simulink model "Expt_2_1"  (R2018a)
settings: Solver=VariableStepAuto  StartTime=0.0  StopTime=10.0  RelTol=1e-3
settings Model: Creator=HP  LastModifiedBy=HP

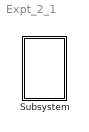
== system Expt_2_1 ==
  Subsystem : Subsystem

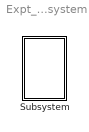
== system Expt_2_1/Subsystem ==
  Subsystem : Subsystem

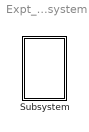
== system Expt_2_1/Subsystem/Subsystem ==
  Subsystem : Subsystem

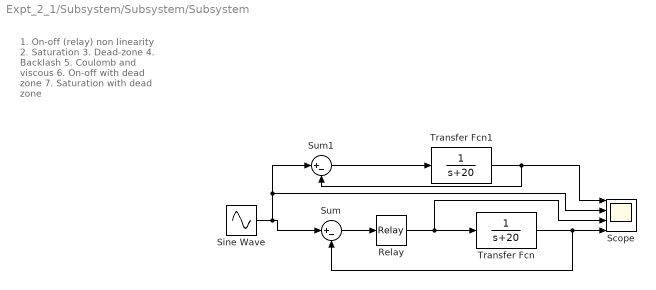
== system Expt_2_1/Subsystem/Subsystem/Subsystem ==
  note: 1. On-off (relay) non linearity
      | 2. Saturation
      | 3. Dead-zone
      | 4. Backlash
      | 5. Coulomb and viscous
      | 6. On-off with dead zone
      | 7. Saturation with dead zone
  Relay : Relay
  Scope : Scope  NumInputPorts=4
  Sine Wave : Sin  SampleTime=0
  Sum : Sum  Inputs=|+-
  Sum1 : Sum  Inputs=|+-
  Transfer Fcn : TransferFcn  Denominator=[1 20]
  Transfer Fcn1 : TransferFcn  Denominator=[1 20]
  wires:
  Sum1/1 -> Transfer Fcn1/1
  Sum/1 -> Relay/1
  Sine Wave/1 -> Sum/1, Scope/2, Sum1/1
  Relay/1 -> Scope/3, Transfer Fcn/1
  Transfer Fcn1/1 -> Scope/1, Sum1/2
  Transfer Fcn/1 -> Scope/4, Sum/2
